simulink model "CrazyFlie"  (R2024a)
settings: Solver=FixedStepAuto  StartTime=0.0  StopTime=8  FixedStep=0.002  RelTol=1e-3
undefined symbols (not defined in the file): Estimatex, Estimatey, Estimatez
libraries: uavsim3dlib x3, simulink_extras x2, sim3dlib x1
settings Model: SnapshotInterval=1  Creator=Guy  LastModifiedBy=User
settings OptimizationCC: ReuseModelBlockBuffer=off
settings ModelReferenceCC: EnableRefExpFcnMdlSchedulingChecks=on
settings RTWCC: GPUComputeCapability=3.5

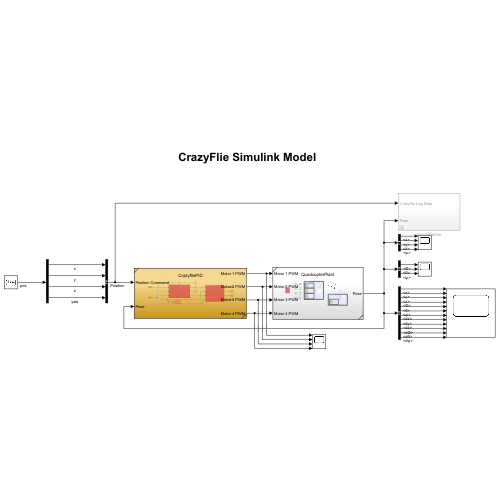
[thumbnail: Simulink's stored preview of the top-level diagram]
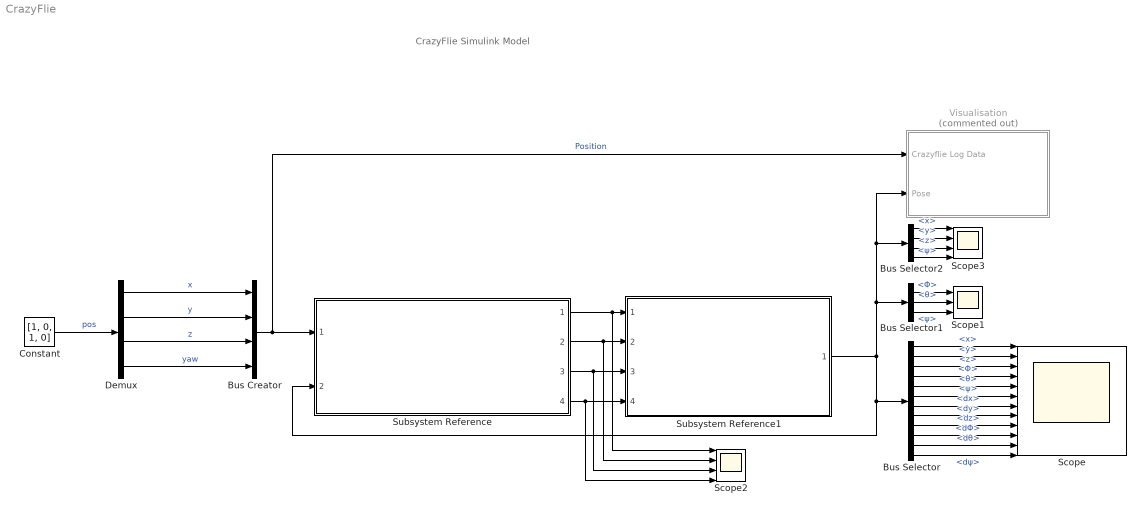
== system CrazyFlie ==
  note: CrazyFlie Simulink Model
  Bus Creator : BusCreator  Inputs=4
  Bus Selector : BusSelector  OutputSignals=Position State.position.x,Position State.position.y,Position State.position.z,Attitude State.attitude.Φ,Attitude State.attitude.θ,Attitude State.attitude.ψ,Position State.velocity.dx,Position State.velocity.dy,Position State.velocity.dz,Attitude State.attitude rate.dΦ,Attitude State.attitude rate.dθ,Attitude State.attitude rate.dψ
  Bus Selector1 : BusSelector  OutputSignals=Attitude State.attitude.Φ,Attitude State.attitude.θ,Attitude State.attitude.ψ
  Bus Selector2 : BusSelector  OutputSignals=Position State.position.x,Position State.position.y,Position State.position.z,Attitude State.attitude.ψ
  Constant : Constant  Value=[1, 0, 1, 0]  VectorParams1D=off
  Demux : Demux
  Scope : Scope  NumInputPorts=12
  Scope1 : Scope  NumInputPorts=3
  Scope2 : Scope  NumInputPorts=4
  Scope3 : Scope  NumInputPorts=4
  Subsystem Reference : Subsystem  ReferencedSubsystem=CrazyfliePID
  Subsystem Reference1 : Subsystem  ReferencedSubsystem=QuadcopterPlant
  Visualisation : Subsystem  Commented=on
  wires:
  Bus Creator/1 -> Visualisation/1(Crazyflie Log Data), Subsystem Reference/1  "Position"
  Subsystem Reference/1 -> Subsystem Reference1/1, Scope2/1
  Subsystem Reference/2 -> Subsystem Reference1/2, Scope2/2
  Subsystem Reference/3 -> Subsystem Reference1/3, Scope2/3
  Subsystem Reference/4 -> Subsystem Reference1/4, Scope2/4
  Constant/1 -> Demux/1  "pos"
  Demux/3 -> Bus Creator/3  "z"
  Demux/4 -> Bus Creator/4  "yaw"
  Demux/1 -> Bus Creator/1  "x"
  Bus Selector1/1 -> Scope1/1  "<Φ>"
  Bus Selector1/2 -> Scope1/2  "<θ>"
  Bus Selector1/3 -> Scope1/3  "<ψ>"
  Bus Selector2/1 -> Scope3/1  "<x>"
  Bus Selector2/2 -> Scope3/2  "<y>"
  Bus Selector2/3 -> Scope3/3  "<z>"
  Demux/2 -> Bus Creator/2  "y"
  Bus Selector2/4 -> Scope3/4  "<ψ>"
  Subsystem Reference1/1 -> Visualisation/2(Pose), Bus Selector2/1, Bus Selector1/1, Subsystem Reference/2, Bus Selector/1
  Bus Selector/1 -> Scope/1  "<x>"
  Bus Selector/2 -> Scope/2  "<y>"
  Bus Selector/3 -> Scope/3  "<z>"
  Bus Selector/4 -> Scope/4  "<Φ>"
  Bus Selector/5 -> Scope/5  "<θ>"
  Bus Selector/6 -> Scope/6  "<ψ>"
  Bus Selector/7 -> Scope/7  "<dx>"
  Bus Selector/8 -> Scope/8  "<dy>"
  Bus Selector/9 -> Scope/9  "<dz>"
  Bus Selector/10 -> Scope/10  "<dΦ>"
  Bus Selector/11 -> Scope/11  "<dθ>"
  Bus Selector/12 -> Scope/12  "<dψ>"

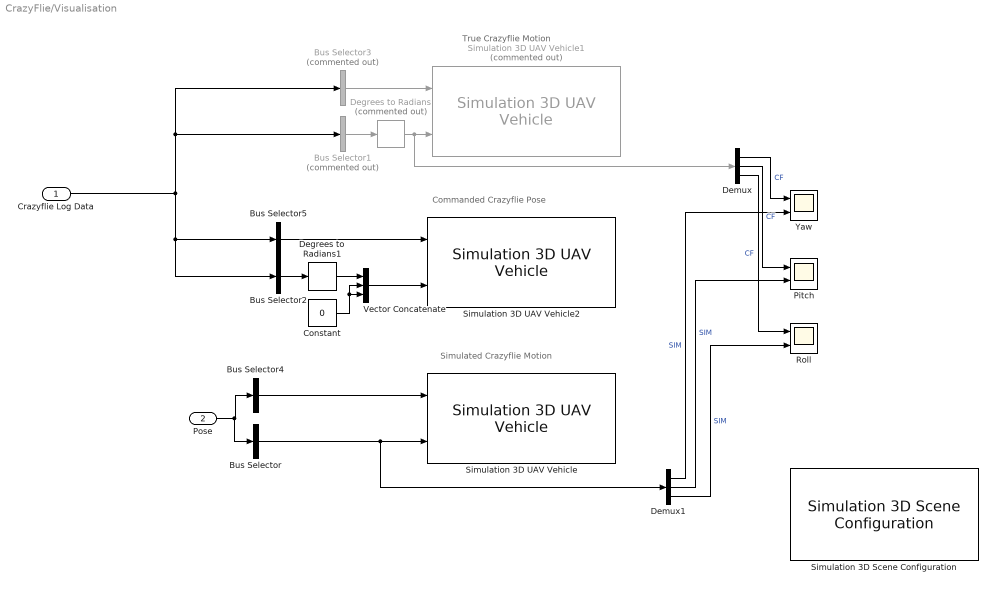
== system CrazyFlie/Visualisation ==
  note: True Crazyflie Motion
  note: Commanded Crazyflie Pose
  note: Simulated Crazyflie Motion
  Crazyflie Log Data : Inport
  Pose : Inport  Port=2
  Bus Selector : BusSelector  OutputSignals=Attitude State.attitude.ψ,Attitude State.attitude.θ,Attitude State.attitude.Φ  OutputAsBus=on
  Bus Selector1 : BusSelector  Commented=on  OutputSignals=EstimateYaw,EstimatePitch,EstimateRoll  OutputAsBus=on
  Bus Selector2 : BusSelector  OutputSignals=yaw  OutputAsBus=on
  Bus Selector3 : BusSelector  Commented=on  OutputSignals=Estimatex,Estimatey,Estimatez  OutputAsBus=on
  Bus Selector4 : BusSelector  OutputSignals=Position State.position.x,Position State.position.y,Position State.position.z  OutputAsBus=on
  Bus Selector5 : BusSelector  OutputSignals=x,y,z  OutputAsBus=on
  Constant : Constant  Value=0
  Degrees to Radians : simulink_extras/Transformations/Degrees to Radians  Commented=on
  Degrees to Radians1 : simulink_extras/Transformations/Degrees to Radians
  Demux : Demux  Outputs=3
  Demux1 : Demux  Outputs=3
  Pitch : Scope  NumInputPorts=2
  Roll : Scope  NumInputPorts=2
  Simulation 3D Scene Configuration : sim3dlib/Simulation 3D Scene Configuration  Priority=0  ProjectFormat=Default Scenes  SceneDesc=US city block  ProjectName=C:\Program Files\MATLAB\R2024a\toolbox\shared\sim3d_projects\automotive_project_windows\UE\WindowsNoEditor\VehicleSimulation.exe  ScenePath=/Game/Maps/USCityBlock  EnableOpenDRIVE=off  vehTagList={'Custom';'Scene Origin';'SimulinkVehicle1';'SimulinkVehicle2';'SimulinkVehicle3'}  vehTag=Custom  FreeCameraInitialTranslation=[-2, 1.5, 1.5]  FreeCameraDefaultInitialTranslation=[-6, 0, 2]  FreeCameraInitialRotation=[0, -10, -30]  FreeCameraDefaultInitialRotation=[0, -15, 0]  OpVisEn=off  Ts=0.03  EnableWindow=on  EnableRemoteAccess=off  EnableWeather=off  SunAzimuth=90  SunAltitude=40.0  EnableGeospatialSun=off  Latitude=0  Longitude=0  Date=2023-01-01  Time=10:30:00  GeoTimeZone=-5.0  SunDaylightSaving=off  wind=1  clouds=10  EnableVolumetricClouds=off  CloudCoverage=0  CloudAltitude=6  fog=0  rain=0  RaindropsEffect=off  SnowDensity=0  EnableGeospatial=off  UseTrueOrigin=off  OriginHeight=200  OriginLatitude=40.744652  OriginLongitude=-73.988864  MapStyle=Aerial  AdditionalAssetIDs=[]  UseAdvancedSunSky=off  SolarTime=11  TimeZone=-5  Day=21  Month=9  Year=2022  UseDaylightSavingTime=on  DSTStartDay=10  DSTStartMonth=3  DSTEndDay=3  DSTEndMonth=11  DSTSwitchHour=2  sensorTag=MainCamera1  sensorId=1  sensorName=MainCamera1  mountLoc=Origin  offsetFlag=off  tmountOffset=[0, 0, 0]  rmountOffset=[0, 0, 0]  HorizontalResolution=1280  VerticalResolution=720  HorizontalFOV=60  mountPoint=[0 0 0]  mountOrientation=[0 0 0]  aMode=4  ID=1  GeoTrigger=Inactive
      settings: LibrarySourceBlock=uavsim3dlib/Simulation 3D Scene Configuration
  Simulation 3D UAV Vehicle : uavsim3dlib/Simulation 3D UAV Vehicle  Priority=-1  Mesh=Quadrotor  MeshPath=/MathWorksUAVContent/UAVs/HexaRotorUAV/HexaRotor.HexaRotor  Color=Black  ActorName=SimulinkVehicle1  UseGlobalFrame=off  InitialTranslation=[0 0 0]  InitialRotation=[0 0 0]  InitialTranslationGlobal=[0 0 0]  InitialGeoOrigin=[0 0 0]  InitialRotationGlobal=[0 0 0]  SampleTime=-1  ActorType=SimulinkVehicle  ID=1  aMode=4  ActorTag=SimulinkVehicle1
  Simulation 3D UAV Vehicle1 : uavsim3dlib/Simulation 3D UAV Vehicle  Priority=-1  Commented=on  Mesh=Quadrotor  MeshPath=/MathWorksUAVContent/UAVs/HexaRotorUAV/HexaRotor.HexaRotor  Color=Green  ActorName=SimulinkVehicle2  UseGlobalFrame=off  InitialTranslation=[Estimatex(1,2) Estimatey(1,2) Estimatez(1,2)]  InitialRotation=[0 0 0]  InitialTranslationGlobal=[0 0 0]  InitialGeoOrigin=[0 0 0]  InitialRotationGlobal=[0 0 0]  SampleTime=-1  ActorType=SimulinkVehicle  ID=2  aMode=4  ActorTag=SimulinkVehicle2
  Simulation 3D UAV Vehicle2 : uavsim3dlib/Simulation 3D UAV Vehicle  Priority=-1  Mesh=Quadrotor  MeshPath=/MathWorksUAVContent/UAVs/HexaRotorUAV/HexaRotor.HexaRotor  Color=Black  ActorName=SimulinkVehicle3  UseGlobalFrame=off  InitialTranslation=[0 0 0]  InitialRotation=[0 0 0]  InitialTranslationGlobal=[0 0 0]  InitialGeoOrigin=[0 0 0]  InitialRotationGlobal=[0 0 0]  SampleTime=-1  ActorType=SimulinkVehicle  ID=3  aMode=4  ActorTag=SimulinkVehicle3
  Vector Concatenate : Concatenate  NumInputs=3
  Yaw : Scope  NumInputPorts=2
  wires:
  Crazyflie Log Data/1 -> Bus Selector5/1, Bus Selector2/1, Bus Selector3/1, Bus Selector1/1
  Degrees to Radians/1 -> Demux/1, Simulation 3D UAV Vehicle1/2
  Bus Selector/1 -> Demux1/1, Simulation 3D UAV Vehicle/2
  Bus Selector3/1 -> Simulation 3D UAV Vehicle1/1
  Bus Selector5/1 -> Simulation 3D UAV Vehicle2/1
  Bus Selector1/1 -> Degrees to Radians/1
  Bus Selector2/1 -> Degrees to Radians1/1
  Pose/1 -> Bus Selector/1, Bus Selector4/1
  Demux/1 -> Yaw/1  "CF"
  Demux1/1 -> Yaw/2  "SIM"
  Demux/2 -> Pitch/1  "CF"
  Demux1/2 -> Pitch/2  "SIM"
  Demux/3 -> Roll/1  "CF"
  Demux1/3 -> Roll/2  "SIM"
  Bus Selector4/1 -> Simulation 3D UAV Vehicle/1
  Degrees to Radians1/1 -> Vector Concatenate/1
  Constant/1 -> Vector Concatenate/2, Vector Concatenate/3
  Vector Concatenate/1 -> Simulation 3D UAV Vehicle2/2
